simulink model "prac2s2022a"  (R2022a)
settings: Solver=FixedStepAuto  StartTime=0.0  StopTime=Tmdl  FixedStep=1e-4  RelTol=1e-3
undefined symbols (not defined in the file): J_sigma, K, Ka, Kc, kc, kd, ke, Kf, km, Komega, Ktheta, na, Tc, Te_val, Tl, Tm
settings Model: Creator=86156  LastModifiedBy=86156
settings ModelReferenceCC: EnableRefExpFcnMdlSchedulingChecks=off
settings RTWCC: Description=Generic Real-Time Target  GPUComputeCapability=5.0

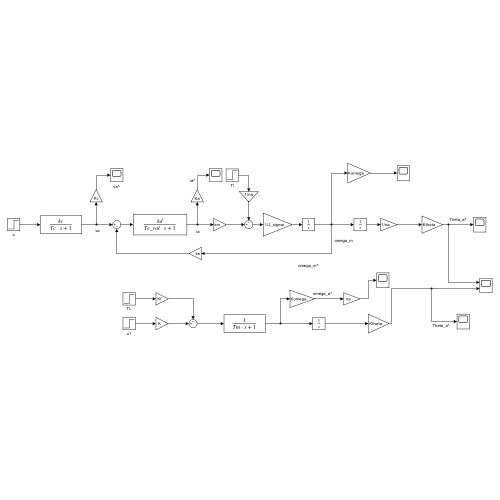
[thumbnail: Simulink's stored preview of the top-level diagram]
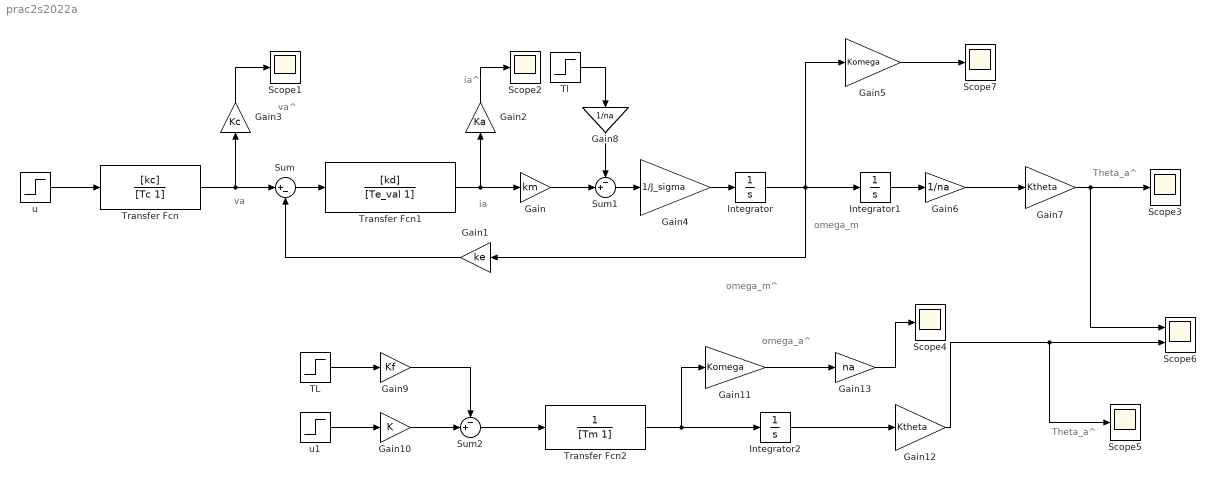
== system prac2s2022a ==
  note: omega_a^
  note: Theta_a^
  note: omega_m
  note: ia
  note: va
  note: va^
  note: ia^
  note: omega_m^
  note: Theta_a^
  Gain : Gain  Gain=km
  Gain1 : Gain  Gain=ke
  Gain10 : Gain  Gain=K
  Gain11 : Gain  Gain=Komega
  Gain12 : Gain  Gain=Ktheta
  Gain13 : Gain  Gain=na
  Gain2 : Gain  Gain=Ka
  Gain3 : Gain  Gain=Kc
  Gain4 : Gain  Gain=1/J_sigma
  Gain5 : Gain  Gain=Komega
  Gain6 : Gain  Gain=1/na
  Gain7 : Gain  Gain=Ktheta
  Gain8 : Gain  Gain=1/na
  Gain9 : Gain  Gain=Kf
  Integrator : Integrator
  Integrator1 : Integrator
  Integrator2 : Integrator
  Scope{1..5,7} (6 alike) : Scope
  Scope6 : Scope  NumInputPorts=2
  Sum : Sum  Inputs=|+-
  Sum1 : Sum  Inputs=-+|
  Sum2 : Sum  Inputs=-+|
  TL : Step  Time=0  After=Tl  SampleTime=0
  Tl : Step  Time=0  After=Tl  SampleTime=0
  Transfer Fcn : TransferFcn  Numerator=[kc]  Denominator=[Tc 1]
  Transfer Fcn1 : TransferFcn  Numerator=[kd]  Denominator=[Te_val 1]
  Transfer Fcn2 : TransferFcn  Denominator=[Tm 1]
  u : Step  Time=0  After=u  SampleTime=0
  u1 : Step  Time=0  After=u  SampleTime=0
  wires:
  u/1 -> Transfer Fcn/1
  Transfer Fcn/1 -> Gain3/1, Sum/1
  Sum/1 -> Transfer Fcn1/1
  Transfer Fcn1/1 -> Gain2/1, Gain/1
  Gain/1 -> Sum1/2
  Gain1/1 -> Sum/2
  Tl/1 -> Gain8/1
  Sum1/1 -> Gain4/1
  Gain4/1 -> Integrator/1
  Integrator/1 -> Gain1/1, Gain5/1, Integrator1/1
  Integrator1/1 -> Gain6/1
  Gain3/1 -> Scope1/1
  Gain2/1 -> Scope2/1
  Gain8/1 -> Sum1/1
  TL/1 -> Gain9/1
  Gain10/1 -> Sum2/2
  Gain9/1 -> Sum2/1
  u1/1 -> Gain10/1
  Sum2/1 -> Transfer Fcn2/1
  Transfer Fcn2/1 -> Integrator2/1, Gain11/1
  Integrator2/1 -> Gain12/1
  Gain6/1 -> Gain7/1
  Gain5/1 -> Scope7/1
  Gain7/1 -> Scope3/1, Scope6/1
  Gain11/1 -> Gain13/1
  Gain12/1 -> Scope5/1, Scope6/2
  Gain13/1 -> Scope4/1
